simulink model "Main_Base_code"  (R2018a)
settings: Solver=VariableStepAuto  StartTime=0.0  StopTime=4  RelTol=1e-3
undefined symbols (not defined in the file): Ion, Lithium
libraries: powerlib x39, electricdrivelib x4, powerlib_meascontrol x2, powerlib_extras x2, simulink x1, re_lib x1
(part 2 of 2)

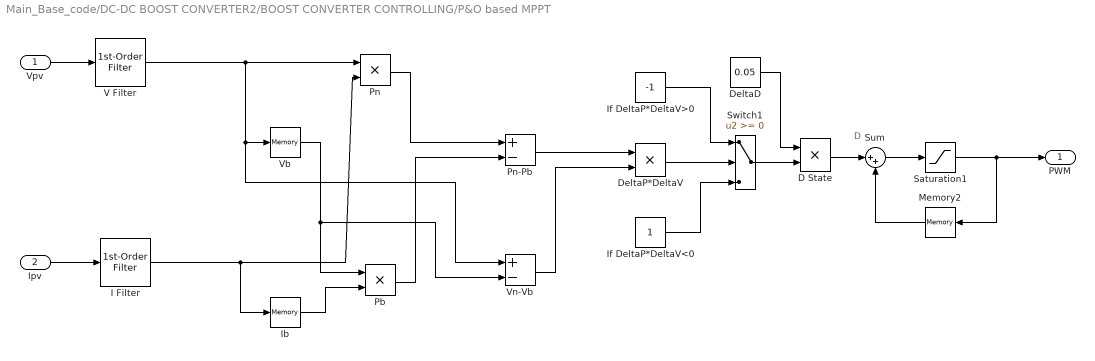
== system Main_Base_code/DC-DC BOOST CONVERTER2/BOOST CONVERTER CONTROLLING/P&O based MPPT ==
  note: D
  Vpv : Inport
  Ipv : Inport  Port=2
  D State : Product  RndMeth=Zero
  DeltaD : Constant  Value=0.05
  DeltaP*DeltaV : Product  RndMeth=Zero
  I Filter : powerlib_extras/Control  Blocks/1st-Order  Filter  FilterType=Lowpass  Tc=1e-3  Initialize=off  Vac_Init=[0.8 -25 60]  Vdc_Init=-0.4  PlotResponse=off  param1=[1 500 1]
  Ib : Memory  InheritSampleTime=on  LinearizeAsDelay=on
  If DeltaP*DeltaV<0 : Constant
  If DeltaP*DeltaV>0 : Constant  Value=-1
  Memory2 : Memory  InheritSampleTime=on
  Pb : Product  RndMeth=Zero
  Pn : Product  RndMeth=Zero
  Pn-Pb : Sum  Inputs=+-
  Saturation1 : Saturate  UpperLimit=0.9  LowerLimit=0.7
  Sum : Sum  Inputs=|++
  Switch1 : Switch
  V Filter : powerlib_extras/Control  Blocks/1st-Order  Filter  FilterType=Lowpass  Tc=1e-3  Initialize=off  Vac_Init=[0.8 -25 60]  Vdc_Init=-0.4  PlotResponse=off  param1=[1 500 1]
  Vb : Memory  InheritSampleTime=on  LinearizeAsDelay=on
  Vn-Vb : Sum  Inputs=+-
  PWM : Outport
  wires:
  Ipv/1 -> I Filter/1
  If DeltaP*DeltaV<0/1 -> Switch1/3
  Pn/1 -> Pn-Pb/1
  V Filter/1 -> Vn-Vb/1, Vb/1, Pn/1
  Ib/1 -> Pb/2
  DeltaP*DeltaV/1 -> Switch1/2
  Vb/1 -> Vn-Vb/2, Pb/1
  If DeltaP*DeltaV>0/1 -> Switch1/1
  Pn-Pb/1 -> DeltaP*DeltaV/1
  Vn-Vb/1 -> DeltaP*DeltaV/2
  I Filter/1 -> Pn/2, Ib/1
  Vpv/1 -> V Filter/1
  Pb/1 -> Pn-Pb/2
  Switch1/1 -> D State/2
  DeltaD/1 -> D State/1
  D State/1 -> Sum/1
  Sum/1 -> Saturation1/1
  Memory2/1 -> Sum/2
  Saturation1/1 -> PWM/1, Memory2/1

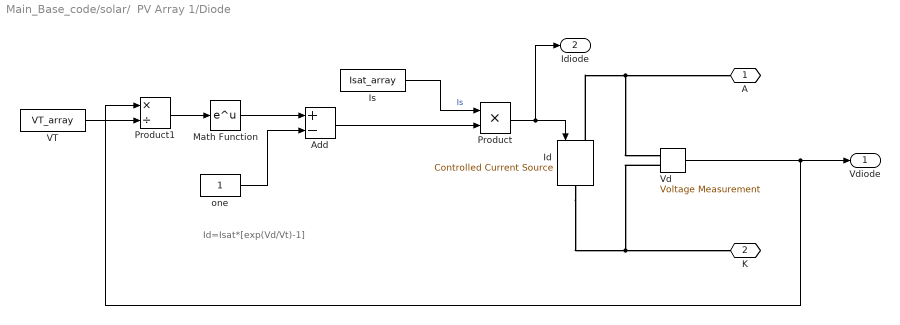
== system Main_Base_code/solar/  PV Array 1/Diode ==
  note: Id=Isat*[exp(Vd/Vt)-1]
  Add : Sum  Inputs=+-
  Id : powerlib/Electrical Sources/Controlled Current Source  Initialize=on  Source_Type=AC  Amplitude=0  Phase=0  Frequency=0  Measurements=None
  Is : Constant  Value=Isat_array
  Math Function : Math  SaturateOnIntegerOverflow=on
  Product : Product  RndMeth=Zero
  Product1 : Product  Inputs=*/  RndMeth=Zero
  VT : Constant  Value=VT_array
  Vd : powerlib/Measurements/Voltage Measurement  PhasorSimulation=off  OutputType=Complex  PSBequivalent=0
  one : Constant
  A : PMIOPort  Side=Left
  K : PMIOPort  Port=2  Side=Right
  Vdiode : Outport
  Idiode : Outport  Port=2
  wires:
  VT/1 -> Product1/2
  Add/1 -> Product/2
  one/1 -> Add/2
  Product1/1 -> Math Function/1
  Is/1 -> Product/1  "Is"
  Vd/1 -> Vdiode/1, Product1/1
  Product/1 -> Id/1, Idiode/1
  Math Function/1 -> Add/1
  connections:
  Id/LConn1 -- A/RConn1 -- Vd/LConn1
  Vd/LConn2 -- K/RConn1 -- Id/RConn1
